simulink model "fullModelKeyboard"  (Simulink 10.0)
settings: Solver=ode23tb  StartTime=0.0  StopTime=1000.0  MaxStep=1  RelTol=1e-3  EnableMultiTasking=on
libraries: LemmingToolbox x11
settings Model: Creator=langmo  LastModifiedBy=unknown
settings DataIOCC: LimitDataPoints=on  SignalLoggingSaveFormat=ModelDataLogs
settings OptimizationCC: ExpressionDepthLimit=2147483647  InitFltsAndDblsToZero=on
settings DebuggingCC: SolverPrmCheckMsg=warning  FcnCallInpInsideContextMsg=warning  StateNameClashWarn=warning
settings SFSimCC: SimUseLocalCustomCode=on  CustomCodeUndefinedFunction=FilterOut
settings RTWCC: RTWUseLocalCustomCode=on

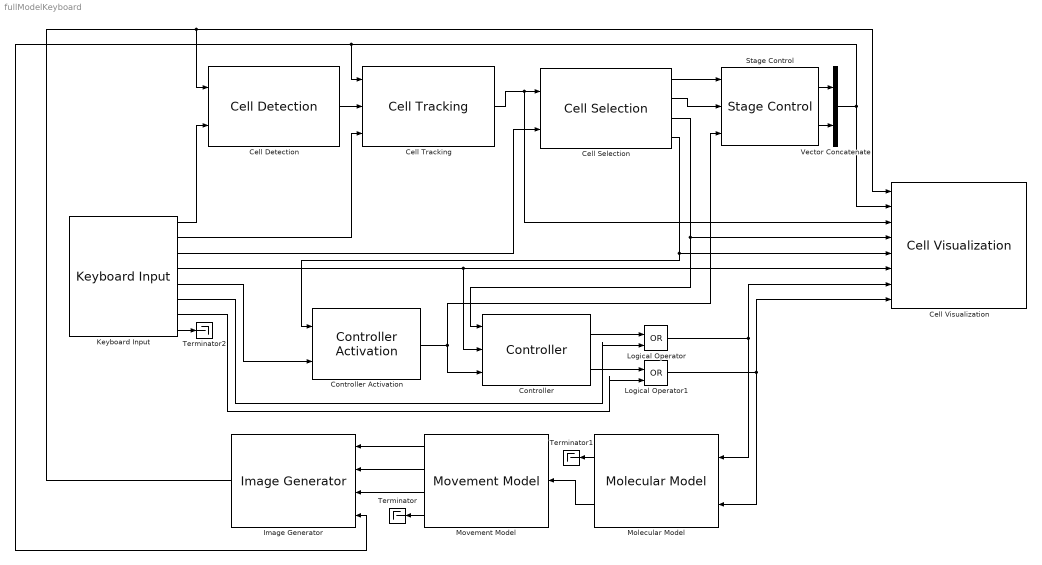
== system fullModelKeyboard ==
  Cell Detection : LemmingToolbox/Cell Detection  SystemSampleTime=-1  imageDim=[1344,1024]  binning=2  cellSizeLowerLimit=70  cellSizeUpperLimit=2000  maxNumCells=1000  resizeScale=0.5  sampleTimes=[0.3, 0.1]
  Cell Selection : LemmingToolbox/Cell Selection  SystemSampleTime=-1  numFrames=2  maxNumCells=1000  sampleTimes=[0.3, 0.1]
  Cell Tracking : LemmingToolbox/Cell Tracking  SystemSampleTime=-1  maxDistance=0.1  maxNumCells=1000  tKeepLost=4  sampleTimes=[0.3, 0.1]
  Cell Visualization : LemmingToolbox/Cell Visualization  SystemSampleTime=-1  outputFilename=fullModel.avi  imageDim=[1344,1024]  binning=2  maxNumCells=1000  coneWidth=150  coneAngle=pi/4  pathLength=30  sampleTimes=[0.3, 0.1]
  Controller : LemmingToolbox/Controller  sampleTimes=[0.3, 0.1]  controller=@controllerHysteresis
  Controller Activation : LemmingToolbox/Controller Activation  SystemSampleTime=-1  isOn=off
  Image Generator : LemmingToolbox/Image Generator  binning=2  numCells=1  sampleTime=[0.3, 0.1]
  Keyboard Input : LemmingToolbox/Keyboard Input  SystemSampleTime=1  initThreshold=0.015  sampleTimes=[0.3, 0.1]
  Logical Operator : Logic  Operator=OR  IconShape=distinctive  AllPortsSameDT=off  OutDataTypeStr=boolean
  Logical Operator1 : Logic  Operator=OR  IconShape=distinctive  AllPortsSameDT=off  OutDataTypeStr=boolean
  Molecular Model : LemmingToolbox/Molecular Model  molecModel=Spiro  controlledCheSpecies=CheY  cheSpeciesAttachedTo=CheX-PhyB & PIF3-Anker  asp=1e-3  useOrgParameters=on  CheX=20  AnkerProt=50  Anker=65
  Movement Model : LemmingToolbox/Movement Model  imageDim=[1344,1024]  binning=2  pixelSize=6.45 / 40  initialCondition=[0.5, 0.5, 0]  sampleTimes=[0.03, 0]
  Stage Control : LemmingToolbox/Stage Control  SystemSampleTime=-1  activate=on  controlMicroscope=off  cooldown=2  border=0.25  initialCondition=[0, 0]  sampleTimes=[0.3, 0.1]
  Terminator : Terminator
  Terminator1 : Terminator
  Terminator2 : Terminator
  Vector Concatenate : Concatenate  ConcatenateDimension=2
  wires:
  Cell Selection/3 -> Cell Visualization/4, Controller/1
  Stage Control/2 -> Vector Concatenate/2
  Stage Control/1 -> Vector Concatenate/1
  Cell Tracking/1 -> Cell Selection/1, Cell Visualization/3
  Cell Detection/1 -> Cell Tracking/2
  Vector Concatenate/1 -> Cell Visualization/2, Cell Tracking/1, Image Generator/4
  Cell Selection/1 -> Stage Control/1
  Cell Selection/2 -> Stage Control/2
  Keyboard Input/1 -> Cell Detection/2
  Keyboard Input/2 -> Cell Tracking/3
  Keyboard Input/3 -> Cell Selection/2
  Controller Activation/1 -> Controller/3, Stage Control/3
  Controller/1 -> Logical Operator/1
  Controller/2 -> Logical Operator1/1
  Keyboard Input/5 -> Controller Activation/2
  Keyboard Input/6 -> Logical Operator/2
  Keyboard Input/7 -> Logical Operator1/2
  Logical Operator/1 -> Molecular Model/1, Cell Visualization/7
  Logical Operator1/1 -> Molecular Model/2, Cell Visualization/8
  Molecular Model/2 -> Movement Model/1
  Molecular Model/1 -> Terminator1/1
  Movement Model/1 -> Image Generator/1
  Movement Model/2 -> Image Generator/2
  Movement Model/3 -> Image Generator/3
  Movement Model/4 -> Terminator/1
  Image Generator/1 -> Cell Visualization/1, Cell Detection/1
  Cell Selection/4 -> Cell Visualization/5, Controller Activation/1
  Keyboard Input/4 -> Controller/2, Cell Visualization/6
  Keyboard Input/8 -> Terminator2/1
